simulink model "Gjennomstrommingsvarme"  (R2025b)
settings: Solver=ode45  StartTime=0.0  StopTime=30  RelTol=1e-3
model workspace (MAT data in the model file):
  SP_Final = 40
  SP_Init = 10
  SP_StepT = 2
  Tin = 10
  q_Final = 12
  q_Init = 8
  q_Lmin = 8
  q_StepT = 15
undefined symbols (not defined in the file): Kd, Ki
libraries: slpidlib x4
settings Model: Creator=Håkon  LastModifiedBy=Håkon

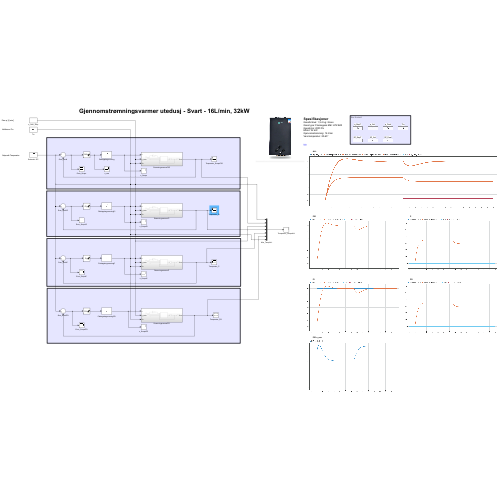
[thumbnail: Simulink's stored preview of the top-level diagram]
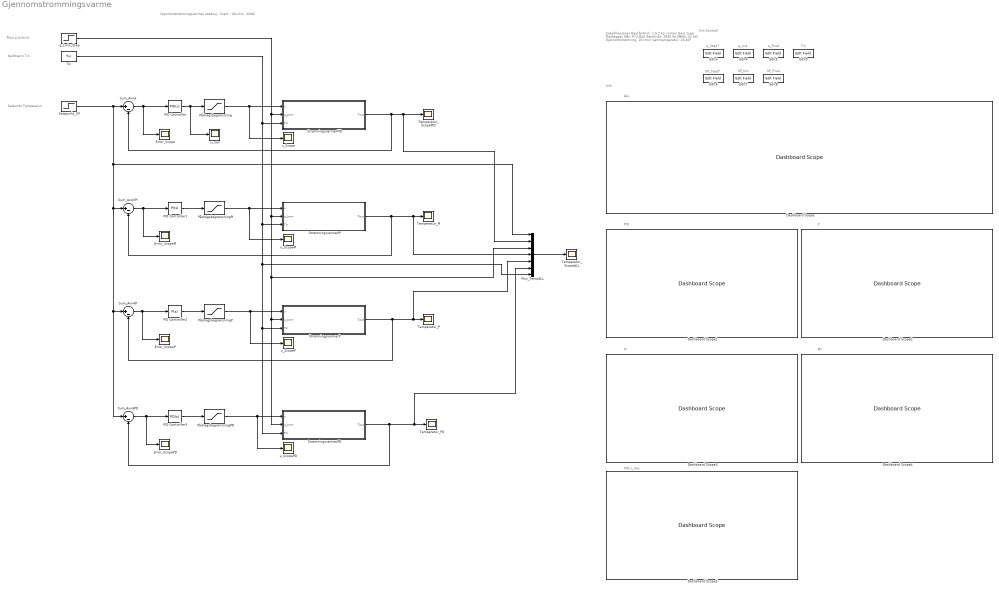
== system Gjennomstrommingsvarme ==
  note: PID
  note: Sim Kontroll
  note: Gjennomstrømningsvarmer utedusj - Svart - 16L/min, 32kW
  note: Spesifikasjoner
      | Gassforbruk: 1,5-2 kg i timen
      | Gass type: Flaskegass Mål: H72:B43
      | Gasstrykk: 2000 Pa
      | Effekt: 32 kW
      | Gjennomstrømning: 16 l/min
      | Vanntemperatur: 20-60°
  note: Link
  note: Kaldtvann Tin
  note: Flow q [L/min]
  note: Setpunkt Temperatur
  note: q_StepT
  note: q_Init
  note: q_Final
  note: SP_StepT
  note: SP_Init
  note: SP_Final
  note: Tin
  note: P
  note: PI
  note: PD
  note: ALL
  note: PID u_raw
  Dashboard Scope{,1..5} (6 alike) : DashboardScope  FontColor=[0.0, 0.0, 0.0]
  Edit{3..9} (7 alike) : EditField  LabelPosition=Hide  ShowInitialText=on  Alignment=Center
  Error_Scope : Scope
      settings: ActiveDisplayYMinimum=-1  ActiveDisplayYMaximum=1
  Error_ScopeP : Scope
      settings: ActiveDisplayYMinimum=-1  ActiveDisplayYMaximum=1  DataLoggingVariableName=ScopeData6
  Error_ScopePD : Scope
      settings: ActiveDisplayYMinimum=-1  ActiveDisplayYMaximum=1  DataLoggingVariableName=ScopeData9
  Error_ScopePI : Scope
      settings: ActiveDisplayYMinimum=-1  ActiveDisplayYMaximum=1  DataLoggingVariableName=ScopeData3
  Mux_TempALL : Mux  Inputs=7
  PID Controller : slpidlib/PID Controller  Controller=PID  Form=Parallel  TimeDomain=Continuous-time  UseExternalTs=off  SampleTime=-1  IntegratorMethod=Forward Euler  FilterMethod=Forward Euler  ControllerParametersSource=internal  P=0.03  I=0.03  UseKiTs=off  D=-0.002  UseExternalDerivativeSource=off  N=2  UseFilter=on  TunerSelectOption=Transfer Function Based (PID Tuner App)  InitialConditionSource=internal  InitialConditionForIntegrator=0  InitialConditionForFilter=0  DifferentiatorICPrevScaledInput=0  ExternalReset=none  TrackingMode=off  Kt=1  LimitOutput=on  SatLimitsSource=internal  UpperSaturationLimit=1  LowerSaturationLimit=0  LinearizeAsGain=on  AntiWindupMode=clamping  Kb=1  LimitIntegrator=off  UpperIntegratorSaturationLimit=inf  LowerIntegratorSaturationLimit=-inf  POutMin=[]  POutMax=[]  IOutMin=[]  IOutMax=[]  DOutMin=[]  DOutMax=[]  NOutMin=[]  NOutMax=[]  SumOutMin=[]  SumOutMax=[]  SaturationOutMin=[]  SaturationOutMax=[]  PParamMin=[]  PParamMax=[]  IParamMin=[]  IParamMax=[]  DParamMin=[]  DParamMax=[]  NParamMin=[]  NParamMax=[]  KbParamMin=[]  KbParamMax=[]  KtParamMin=[]  KtParamMax=[]  KbOutMin=[]  KbOutMax=[]  KtOutMin=[]  KtOutMax=[]  IntegratorOutMin=[]  IntegratorOutMax=[]  FilterOutMin=[]  FilterOutMax=[]  SumI1OutMin=[]  SumI1OutMax=[]  SumI2OutMin=[]  SumI2OutMax=[]  SumI3OutMin=[]  SumI3OutMax=[]  SumI4OutMin=[]  SumI4OutMax=[]  SumDOutMin=[]  SumDOutMax=[]  DifferentiatorOutMin=[]  DifferentiatorOutMax=[]  FilterDiffOutCoefMin=[]  FilterDiffOutCoefMax=[]  ReciprocalOutMin=[]  ReciprocalOutMax=[]  SumDenOutMin=[]  SumDenOutMax=[]  SumNumOutMin=[]  SumNumOutMax=[]  DivideOutMin=[]  DivideOutMax=[]  UdiffTsProdOutMin=[]  UdiffTsProdOutMax=[]  NTsProdOutMin=[]  NTsProdOutMax=[]  UintegralTsProdOutMin=[]  UintegralTsProdOutMax=[]  UngainTsProdOutMin=[]  UngainTsProdOutMax=[]  ClampingZeroOutDataTypeStr=Inherit: Inherit via back propagation  ClampingZeroOutMin=[]  ClampingZeroOutMax=[]  FilterDenConstantOutDataTypeStr=Inherit: Inherit via back propagation  FilterDenConstantOutMin=[]  FilterDenConstantOutMax=[]  PCopyOutDataTypeStr=Inherit: Inherit via back propagation  PCopyOutMin=[]  PCopyOutMax=[]  NCopyOutDataTypeStr=Inherit: Inherit via back propagation  NCopyOutMin=[]  NCopyOutMax=[]  IntegratorContinuousStateAttributes=''  IntegratorStateMustResolveToSignalObject=off  IntegratorRTWStateStorageClass=Auto  FilterContinuousStateAttributes=''  FilterStateMustResolveToSignalObject=off  FilterRTWStateStorageClass=Auto  ParallelPVariant=InternalParameters  IdealPVariant=Disabled  IVariant=InternalParameters  DVariant=InternalParameters  IntegratorVariant=Continuous  SatVariant=Enabled  AWVariant=ContClampingParallel  PCopyVariant=Disabled  TRVariant=Disabled  FdbkBlocksVariant=Forward  IdealPFdbkVariant=Disabled  SatFdbkVariant=Disabled  DerivativeFilterVariant=ContFilter  NVariant=InternalParameters  NCopyVariant=Disabled  FilterICVariant=InternalICsFilter  IntegratorICVariant=InternalICs  ExternalResetVariant=Disabled  TRSumVariant=Passthrough  SumFdbkVariant=Disabled  SumVariant=Sum_PID  TsampFilterVariant=InternalTs  TsampNgainVariant=Passthrough  TsampIntegralVariant=Disabled_SignalSpec  ExternalSaturationOutDataTypeStr=Inherit: Same as second input  DerivativeSourceVariant=ErrorSignal  PreIntVariant=InternalPreInt
  PID Controller1 : slpidlib/PID Controller  Controller=PI  Form=Parallel  TimeDomain=Continuous-time  UseExternalTs=off  SampleTime=-1  IntegratorMethod=Forward Euler  FilterMethod=Forward Euler  ControllerParametersSource=internal  P=0.03  I=0.03  UseKiTs=off  D=Kd  UseExternalDerivativeSource=off  N=100  UseFilter=on  TunerSelectOption=Transfer Function Based (PID Tuner App)  InitialConditionSource=internal  InitialConditionForIntegrator=0  InitialConditionForFilter=0  DifferentiatorICPrevScaledInput=0  ExternalReset=none  TrackingMode=off  Kt=1  LimitOutput=on  SatLimitsSource=internal  UpperSaturationLimit=1  LowerSaturationLimit=0  LinearizeAsGain=on  AntiWindupMode=clamping  Kb=1  LimitIntegrator=off  UpperIntegratorSaturationLimit=inf  LowerIntegratorSaturationLimit=-inf  POutMin=[]  POutMax=[]  IOutMin=[]  IOutMax=[]  DOutMin=[]  DOutMax=[]  NOutMin=[]  NOutMax=[]  SumOutMin=[]  SumOutMax=[]  SaturationOutMin=[]  SaturationOutMax=[]  PParamMin=[]  PParamMax=[]  IParamMin=[]  IParamMax=[]  DParamMin=[]  DParamMax=[]  NParamMin=[]  NParamMax=[]  KbParamMin=[]  KbParamMax=[]  KtParamMin=[]  KtParamMax=[]  KbOutMin=[]  KbOutMax=[]  KtOutMin=[]  KtOutMax=[]  IntegratorOutMin=[]  IntegratorOutMax=[]  FilterOutMin=[]  FilterOutMax=[]  SumI1OutMin=[]  SumI1OutMax=[]  SumI2OutMin=[]  SumI2OutMax=[]  SumI3OutMin=[]  SumI3OutMax=[]  SumI4OutMin=[]  SumI4OutMax=[]  SumDOutMin=[]  SumDOutMax=[]  DifferentiatorOutMin=[]  DifferentiatorOutMax=[]  FilterDiffOutCoefMin=[]  FilterDiffOutCoefMax=[]  ReciprocalOutMin=[]  ReciprocalOutMax=[]  SumDenOutMin=[]  SumDenOutMax=[]  SumNumOutMin=[]  SumNumOutMax=[]  DivideOutMin=[]  DivideOutMax=[]  UdiffTsProdOutMin=[]  UdiffTsProdOutMax=[]  NTsProdOutMin=[]  NTsProdOutMax=[]  UintegralTsProdOutMin=[]  UintegralTsProdOutMax=[]  UngainTsProdOutMin=[]  UngainTsProdOutMax=[]  ClampingZeroOutDataTypeStr=Inherit: Inherit via back propagation  ClampingZeroOutMin=[]  ClampingZeroOutMax=[]  FilterDenConstantOutDataTypeStr=Inherit: Inherit via back propagation  FilterDenConstantOutMin=[]  FilterDenConstantOutMax=[]  PCopyOutDataTypeStr=Inherit: Inherit via back propagation  PCopyOutMin=[]  PCopyOutMax=[]  NCopyOutDataTypeStr=Inherit: Inherit via back propagation  NCopyOutMin=[]  NCopyOutMax=[]  IntegratorContinuousStateAttributes=''  IntegratorStateMustResolveToSignalObject=off  IntegratorRTWStateStorageClass=Auto  FilterContinuousStateAttributes=''  FilterStateMustResolveToSignalObject=off  FilterRTWStateStorageClass=Auto  ParallelPVariant=InternalParameters  IdealPVariant=Disabled  IVariant=InternalParameters  DVariant=Disabled  IntegratorVariant=Continuous  SatVariant=Enabled  AWVariant=ContClampingParallel  PCopyVariant=Disabled  TRVariant=Disabled  FdbkBlocksVariant=Forward  IdealPFdbkVariant=Disabled  SatFdbkVariant=Disabled  DerivativeFilterVariant=Disabled  NVariant=Disabled  NCopyVariant=Disabled_SignalSpec  FilterICVariant=Disabled  IntegratorICVariant=InternalICs  ExternalResetVariant=Disabled  TRSumVariant=Passthrough  SumFdbkVariant=Disabled  SumVariant=Sum_PI  TsampFilterVariant=InternalTs  TsampNgainVariant=Passthrough  TsampIntegralVariant=Disabled_SignalSpec  ExternalSaturationOutDataTypeStr=Inherit: Same as second input  DerivativeSourceVariant=Disabled  PreIntVariant=InternalPreInt
  PID Controller2 : slpidlib/PID Controller  Controller=P  Form=Parallel  TimeDomain=Continuous-time  UseExternalTs=off  SampleTime=-1  IntegratorMethod=Forward Euler  FilterMethod=Forward Euler  ControllerParametersSource=internal  P=0.03  I=Ki  UseKiTs=off  D=Kd  UseExternalDerivativeSource=off  N=100  UseFilter=on  TunerSelectOption=Transfer Function Based (PID Tuner App)  InitialConditionSource=internal  InitialConditionForIntegrator=0  InitialConditionForFilter=0  DifferentiatorICPrevScaledInput=0  ExternalReset=none  TrackingMode=off  Kt=1  LimitOutput=on  SatLimitsSource=internal  UpperSaturationLimit=1  LowerSaturationLimit=0  LinearizeAsGain=on  AntiWindupMode=clamping  Kb=1  LimitIntegrator=off  UpperIntegratorSaturationLimit=inf  LowerIntegratorSaturationLimit=-inf  POutMin=[]  POutMax=[]  IOutMin=[]  IOutMax=[]  DOutMin=[]  DOutMax=[]  NOutMin=[]  NOutMax=[]  SumOutMin=[]  SumOutMax=[]  SaturationOutMin=[]  SaturationOutMax=[]  PParamMin=[]  PParamMax=[]  IParamMin=[]  IParamMax=[]  DParamMin=[]  DParamMax=[]  NParamMin=[]  NParamMax=[]  KbParamMin=[]  KbParamMax=[]  KtParamMin=[]  KtParamMax=[]  KbOutMin=[]  KbOutMax=[]  KtOutMin=[]  KtOutMax=[]  IntegratorOutMin=[]  IntegratorOutMax=[]  FilterOutMin=[]  FilterOutMax=[]  SumI1OutMin=[]  SumI1OutMax=[]  SumI2OutMin=[]  SumI2OutMax=[]  SumI3OutMin=[]  SumI3OutMax=[]  SumI4OutMin=[]  SumI4OutMax=[]  SumDOutMin=[]  SumDOutMax=[]  DifferentiatorOutMin=[]  DifferentiatorOutMax=[]  FilterDiffOutCoefMin=[]  FilterDiffOutCoefMax=[]  ReciprocalOutMin=[]  ReciprocalOutMax=[]  SumDenOutMin=[]  SumDenOutMax=[]  SumNumOutMin=[]  SumNumOutMax=[]  DivideOutMin=[]  DivideOutMax=[]  UdiffTsProdOutMin=[]  UdiffTsProdOutMax=[]  NTsProdOutMin=[]  NTsProdOutMax=[]  UintegralTsProdOutMin=[]  UintegralTsProdOutMax=[]  UngainTsProdOutMin=[]  UngainTsProdOutMax=[]  ClampingZeroOutDataTypeStr=Inherit: Inherit via back propagation  ClampingZeroOutMin=[]  ClampingZeroOutMax=[]  FilterDenConstantOutDataTypeStr=Inherit: Inherit via back propagation  FilterDenConstantOutMin=[]  FilterDenConstantOutMax=[]  PCopyOutDataTypeStr=Inherit: Inherit via back propagation  PCopyOutMin=[]  PCopyOutMax=[]  NCopyOutDataTypeStr=Inherit: Inherit via back propagation  NCopyOutMin=[]  NCopyOutMax=[]  IntegratorContinuousStateAttributes=''  IntegratorStateMustResolveToSignalObject=off  IntegratorRTWStateStorageClass=Auto  FilterContinuousStateAttributes=''  FilterStateMustResolveToSignalObject=off  FilterRTWStateStorageClass=Auto  ParallelPVariant=InternalParameters  IdealPVariant=Disabled  IVariant=Disabled  DVariant=Disabled  IntegratorVariant=Disabled  SatVariant=Enabled  AWVariant=Disabled  PCopyVariant=Disabled  TRVariant=Disabled  FdbkBlocksVariant=Forward  IdealPFdbkVariant=Disabled  SatFdbkVariant=Disabled  DerivativeFilterVariant=Disabled  NVariant=Disabled  NCopyVariant=Disabled_SignalSpec  FilterICVariant=Disabled  IntegratorICVariant=Disabled  ExternalResetVariant=Disabled  TRSumVariant=Passthrough  SumFdbkVariant=Disabled  SumVariant=Passthrough_P  TsampFilterVariant=InternalTs  TsampNgainVariant=Passthrough  TsampIntegralVariant=Disabled_SignalSpec  ExternalSaturationOutDataTypeStr=Inherit: Same as second input  DerivativeSourceVariant=Disabled  PreIntVariant=InternalPreInt
  PID Controller3 : slpidlib/PID Controller  Controller=PD  Form=Parallel  TimeDomain=Continuous-time  UseExternalTs=off  SampleTime=-1  IntegratorMethod=Forward Euler  FilterMethod=Forward Euler  ControllerParametersSource=internal  P=0.03  I=Ki  UseKiTs=off  D=-0.002  UseExternalDerivativeSource=off  N=2  UseFilter=on  TunerSelectOption=Transfer Function Based (PID Tuner App)  InitialConditionSource=internal  InitialConditionForIntegrator=0  InitialConditionForFilter=0  DifferentiatorICPrevScaledInput=0  ExternalReset=none  TrackingMode=off  Kt=1  LimitOutput=on  SatLimitsSource=internal  UpperSaturationLimit=1  LowerSaturationLimit=0  LinearizeAsGain=on  AntiWindupMode=clamping  Kb=1  LimitIntegrator=off  UpperIntegratorSaturationLimit=inf  LowerIntegratorSaturationLimit=-inf  POutMin=[]  POutMax=[]  IOutMin=[]  IOutMax=[]  DOutMin=[]  DOutMax=[]  NOutMin=[]  NOutMax=[]  SumOutMin=[]  SumOutMax=[]  SaturationOutMin=[]  SaturationOutMax=[]  PParamMin=[]  PParamMax=[]  IParamMin=[]  IParamMax=[]  DParamMin=[]  DParamMax=[]  NParamMin=[]  NParamMax=[]  KbParamMin=[]  KbParamMax=[]  KtParamMin=[]  KtParamMax=[]  KbOutMin=[]  KbOutMax=[]  KtOutMin=[]  KtOutMax=[]  IntegratorOutMin=[]  IntegratorOutMax=[]  FilterOutMin=[]  FilterOutMax=[]  SumI1OutMin=[]  SumI1OutMax=[]  SumI2OutMin=[]  SumI2OutMax=[]  SumI3OutMin=[]  SumI3OutMax=[]  SumI4OutMin=[]  SumI4OutMax=[]  SumDOutMin=[]  SumDOutMax=[]  DifferentiatorOutMin=[]  DifferentiatorOutMax=[]  FilterDiffOutCoefMin=[]  FilterDiffOutCoefMax=[]  ReciprocalOutMin=[]  ReciprocalOutMax=[]  SumDenOutMin=[]  SumDenOutMax=[]  SumNumOutMin=[]  SumNumOutMax=[]  DivideOutMin=[]  DivideOutMax=[]  UdiffTsProdOutMin=[]  UdiffTsProdOutMax=[]  NTsProdOutMin=[]  NTsProdOutMax=[]  UintegralTsProdOutMin=[]  UintegralTsProdOutMax=[]  UngainTsProdOutMin=[]  UngainTsProdOutMax=[]  ClampingZeroOutDataTypeStr=Inherit: Inherit via back propagation  ClampingZeroOutMin=[]  ClampingZeroOutMax=[]  FilterDenConstantOutDataTypeStr=Inherit: Inherit via back propagation  FilterDenConstantOutMin=[]  FilterDenConstantOutMax=[]  PCopyOutDataTypeStr=Inherit: Inherit via back propagation  PCopyOutMin=[]  PCopyOutMax=[]  NCopyOutDataTypeStr=Inherit: Inherit via back propagation  NCopyOutMin=[]  NCopyOutMax=[]  IntegratorContinuousStateAttributes=''  IntegratorStateMustResolveToSignalObject=off  IntegratorRTWStateStorageClass=Auto  FilterContinuousStateAttributes=''  FilterStateMustResolveToSignalObject=off  FilterRTWStateStorageClass=Auto  ParallelPVariant=InternalParameters  IdealPVariant=Disabled  IVariant=Disabled  DVariant=InternalParameters  IntegratorVariant=Disabled  SatVariant=Enabled  AWVariant=Disabled  PCopyVariant=Disabled  TRVariant=Disabled  FdbkBlocksVariant=Forward  IdealPFdbkVariant=Disabled  SatFdbkVariant=Disabled  DerivativeFilterVariant=ContFilter  NVariant=InternalParameters  NCopyVariant=Disabled  FilterICVariant=InternalICsFilter  IntegratorICVariant=Disabled  ExternalResetVariant=Disabled  TRSumVariant=Passthrough  SumFdbkVariant=Disabled  SumVariant=Sum_PD  TsampFilterVariant=InternalTs  TsampNgainVariant=Passthrough  TsampIntegralVariant=Disabled_SignalSpec  ExternalSaturationOutDataTypeStr=Inherit: Same as second input  DerivativeSourceVariant=ErrorSignal  PreIntVariant=InternalPreInt
  Pådragsbegrensning : Saturate  UpperLimit=1  LowerLimit=0
  PådragsbegrensningP : Saturate  UpperLimit=1  LowerLimit=0
  PådragsbegrensningPD : Saturate  UpperLimit=1  LowerLimit=0
  PådragsbegrensningPI : Saturate  UpperLimit=1  LowerLimit=0
  Settpunkt_SP : Step  Time=SP_StepT  Before=SP_Init  After=SP_Final  SampleTime=0
  StrømningsvarmerP : Subsystem
  StrømningsvarmerPD : Subsystem
  StrømningsvarmerPI : Subsystem
  StrømningsvarmerPID : Subsystem
  Sum_Avvik : Sum  Inputs=|+-
  Sum_AvvikP : Sum  Inputs=|+-
  Sum_AvvikPD : Sum  Inputs=|+-
  Sum_AvvikPI : Sum  Inputs=|+-
  Temperatur_P : Scope
      settings: ActiveDisplayYMinimum=6.4940957211164019  ActiveDisplayYMaximum=41.55313850995239  DataLoggingVariableName=ScopeData7
  Temperatur_PD : Scope
      settings: ActiveDisplayYMinimum=7.7892303218856442  ActiveDisplayYMaximum=29.89692710302921  DataLoggingVariableName=ScopeData10
  Temperatur_PI : Scope
      settings: ActiveDisplayYMinimum=6.0133689334322051  ActiveDisplayYMaximum=45.879679599110162  DataLoggingVariableName=ScopeData4
  Temperatur_ScopeALL : Scope
      settings: ActiveDisplayYMinimum=-19.252072166409661  ActiveDisplayYMaximum=81.341690384246078  DataLoggingVariableName=ScopeData12
  Temperatur_ScopePID : Scope
      settings: ActiveDisplayYMinimum=6.00522530086716  ActiveDisplayYMaximum=45.952972292195568
  Tin : Constant  Value=Tin
  q_Lmin_Step : Step  Time=q_StepT  Before=q_Init  After=q_Final  SampleTime=0
  u_Scope : Scope
      settings: ActiveDisplayYMinimum=-1  ActiveDisplayYMaximum=1  DataLoggingVariableName=ScopeData2
  u_ScopeP : Scope
      settings: ActiveDisplayYMinimum=-1  ActiveDisplayYMaximum=1  DataLoggingVariableName=ScopeData8
  u_ScopePD : Scope
      settings: ActiveDisplayYMinimum=-1  ActiveDisplayYMaximum=1  DataLoggingVariableName=ScopeData11
  u_ScopePI : Scope
      settings: ActiveDisplayYMinimum=-1  ActiveDisplayYMaximum=1  DataLoggingVariableName=ScopeData5
  u_raw : Scope
      settings: ActiveDisplayYMinimum=-1  ActiveDisplayYMaximum=1  DataLoggingVariableName=ScopeData13
  wires:
  Sum_Avvik/1 -> PID Controller/1, Error_Scope/1
  Pådragsbegrensning/1 -> u_Scope/1, StrømningsvarmerPID/1(u)
  PID Controller/1 -> u_raw/1, Pådragsbegrensning/1
  PådragsbegrensningPI/1 -> StrømningsvarmerPI/1(u), u_ScopePI/1
  Sum_AvvikPI/1 -> PID Controller1/1, Error_ScopePI/1
  StrømningsvarmerPI/1(Tout) -> Mux_TempALL/4, Temperatur_PI/1, Sum_AvvikPI/2
  PID Controller2/1 -> PådragsbegrensningP/1
  StrømningsvarmerP/1(Tout) -> Mux_TempALL/5, Temperatur_P/1, Sum_AvvikP/2
  PådragsbegrensningP/1 -> u_ScopeP/1, StrømningsvarmerP/1(u)
  Sum_AvvikP/1 -> Error_ScopeP/1, PID Controller2/1
  q_Lmin_Step/1 -> Mux_TempALL/3, StrømningsvarmerPD/2(q_Lmin), StrømningsvarmerP/2(q_Lmin), StrømningsvarmerPI/2(q_Lmin), StrømningsvarmerPID/2(q_Lmin)
  Tin/1 -> StrømningsvarmerPID/3(Tin), Mux_TempALL/7, StrømningsvarmerP/3(Tin), StrømningsvarmerPD/3(Tin), StrømningsvarmerPI/3(Tin)
  Settpunkt_SP/1 -> Mux_TempALL/1, Sum_AvvikPI/1, Sum_AvvikPD/1, Sum_AvvikP/1, Sum_Avvik/1
  PID Controller3/1 -> PådragsbegrensningPD/1
  StrømningsvarmerPD/1(Tout) -> Mux_TempALL/6, Temperatur_PD/1, Sum_AvvikPD/2
  PådragsbegrensningPD/1 -> StrømningsvarmerPD/1(u), u_ScopePD/1
  Mux_TempALL/1 -> Temperatur_ScopeALL/1
  Sum_AvvikPD/1 -> Error_ScopePD/1, PID Controller3/1
  PID Controller1/1 -> PådragsbegrensningPI/1
  StrømningsvarmerPID/1(Tout) -> Mux_TempALL/2, Temperatur_ScopePID/1, Sum_Avvik/2

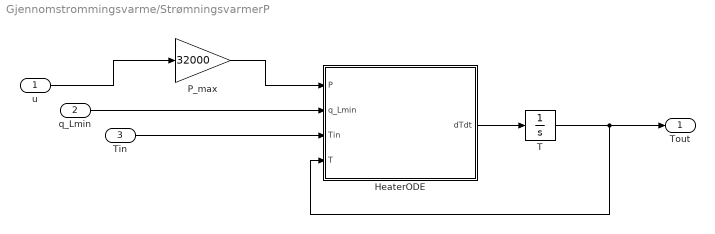
== system Gjennomstrommingsvarme/StrømningsvarmerP ==
  u : Inport
  q_Lmin : Inport  Port=2
  Tin : Inport  Port=3
  HeaterODE : MATLAB Function  TreatAsAtomicUnit=on
  P_max : Gain  Gain=32000
  T : Integrator  InitialCondition=Tin
  Tout : Outport
  wires:
  q_Lmin/1 -> HeaterODE/2(q_Lmin)
  Tin/1 -> HeaterODE/3(Tin)
  HeaterODE/1(dTdt) -> T/1
  T/1 -> Tout/1, HeaterODE/4(T)
  P_max/1 -> HeaterODE/1(P)
  u/1 -> P_max/1

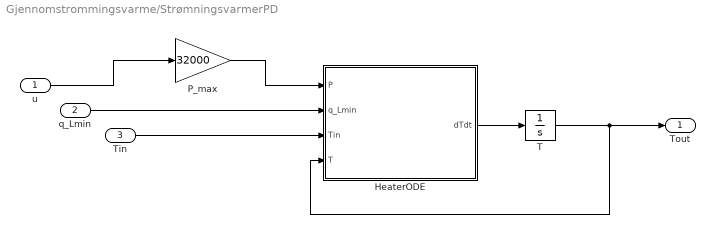
== system Gjennomstrommingsvarme/StrømningsvarmerPD ==
  u : Inport
  q_Lmin : Inport  Port=2
  Tin : Inport  Port=3
  HeaterODE : MATLAB Function  TreatAsAtomicUnit=on
  P_max : Gain  Gain=32000
  T : Integrator  InitialCondition=Tin
  Tout : Outport
  wires:
  q_Lmin/1 -> HeaterODE/2(q_Lmin)
  Tin/1 -> HeaterODE/3(Tin)
  HeaterODE/1(dTdt) -> T/1
  T/1 -> Tout/1, HeaterODE/4(T)
  P_max/1 -> HeaterODE/1(P)
  u/1 -> P_max/1

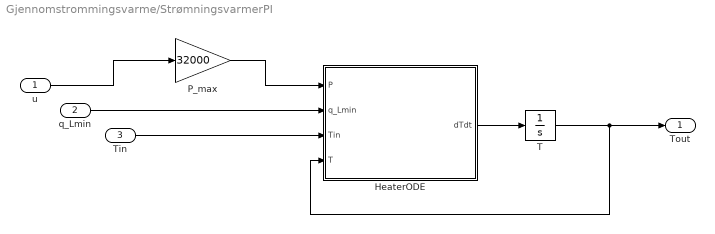
== system Gjennomstrommingsvarme/StrømningsvarmerPI ==
  u : Inport
  q_Lmin : Inport  Port=2
  Tin : Inport  Port=3
  HeaterODE : MATLAB Function  TreatAsAtomicUnit=on
  P_max : Gain  Gain=32000
  T : Integrator  InitialCondition=Tin
  Tout : Outport
  wires:
  q_Lmin/1 -> HeaterODE/2(q_Lmin)
  Tin/1 -> HeaterODE/3(Tin)
  HeaterODE/1(dTdt) -> T/1
  T/1 -> Tout/1, HeaterODE/4(T)
  P_max/1 -> HeaterODE/1(P)
  u/1 -> P_max/1

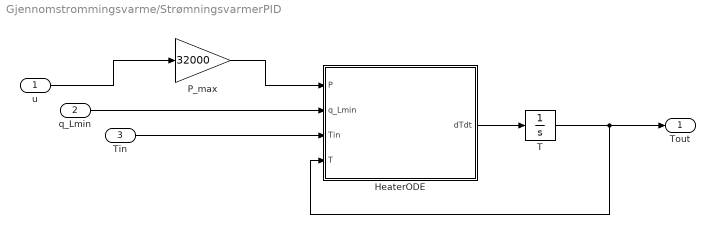
== system Gjennomstrommingsvarme/StrømningsvarmerPID ==
  u : Inport
  q_Lmin : Inport  Port=2
  Tin : Inport  Port=3
  HeaterODE : MATLAB Function  TreatAsAtomicUnit=on
  P_max : Gain  Gain=32000
  T : Integrator  InitialCondition=Tin
  Tout : Outport
  wires:
  q_Lmin/1 -> HeaterODE/2(q_Lmin)
  Tin/1 -> HeaterODE/3(Tin)
  HeaterODE/1(dTdt) -> T/1
  T/1 -> Tout/1, HeaterODE/4(T)
  P_max/1 -> HeaterODE/1(P)
  u/1 -> P_max/1

== matlab function Gjennomstrommingsvarme/StrømningsvarmerPI/HeaterODE ==
  data: P input; dTdt output; q_Lmin input; Tin input; T input
function dTdt = HeaterODE(P, q_Lmin, Tin, T)
% HeaterODE - Forbedret modell for gass-gjennomstroemningsvarmer
% Utendoersdusj 32kW
%
% Denne versjonen bruker SKALAR T (vanntemperatur) slik at den fungerer
% direkte med eksisterende Simulink-modell uten endringer i integrator
% eller signalruting.
%
% Forbedringer vs. original:
%   - Forbrenningsvirkningsgrad (eta = 85%)
%   - Varmetap til omgivelser (UA_ma)
%   - Effektiv varmeovergang justert for gjennomstroemningsvarmer
%
% Referanser:
%   [1] Incropera et al., "Fundamentals of Heat and Mass Transfer", 7e, Wiley, 2011.
%   [2] Cengel, "Heat Transfer: A Practical Approach", 2e, McGraw-Hill, 2003.
%
% Innganger:
%   P       - Varmeeffekt fra brenner [W] (0 til 32000 W)
%   q_Lmin  - Volumstroem vann [L/min] (maks 16 L/min)
%   Tin     - Innloepstemperatur vann [degC]
%   T       - Utloepstemperatur vann [degC] (tilbakekobling, skalar)
%
% Utgang:
%   dTdt    - Temperaturendring [degC/s] (skalar)

% =====================================================================
%  VANNETS EGENSKAPER [1, Tabell A.6]
% =====================================================================
cp    = 4186;          % Spesifikk varmekapasitet vann [J/(kg*K)]
rho   = 1.0;           % Tetthet vann [kg/L]

% =====================================================================
%  FORBRENNINGSEFFEKTIVITET [2, Kap. 13]
% =====================================================================
eta   = 0.85;          % Virkningsgrad gassbrenner (85%)

% =====================================================================
%  MASSESTROEMM
% =====================================================================
mdot  = (q_Lmin / 60) * rho;  % [kg/s]

% =====================================================================
%  VARMEVEKSLER - tilpasset gjennomstroemningsvarmer
% =====================================================================
% Kompakt kobberspiral med direkte flamme.
% Lite vannvolum gir kort oppholdstid (ca. 2 sekunder ved 8 L/min).
V     = 0.25;          % Vannvolum i veksler [L]
C     = V * rho * cp;  % Termisk kapasitet vann [J/K] = 1046.5

% =====================================================================
%  VARMETAP TIL OMGIVELSER
% =====================================================================
UA_loss = 10;          % Konduktans til omgivelser [W/K]
T_amb   = 10;          % Omgivelsestemperatur [degC]
Q_loss  = UA_loss * (T - T_amb);  % Varmetap [W]

% =====================================================================
%  ENERGIBALANSE
% =====================================================================
%  C * dT/dt = eta*P - Q_loss + mdot*cp*(Tin - T)
%
%  Ledd:
%    eta*P              : Effektiv varme fra gassforbrenning [W]
%    Q_loss             : Varmetap til omgivelser [W]
%    mdot*cp*(Tin - T)  : Netto varme fra vannstroemmen [W]

dTdt = (eta * P - Q_loss + mdot * cp * (Tin - T)) / C;

end

== matlab function Gjennomstrommingsvarme/StrømningsvarmerPID/HeaterODE ==
  data: P input; dTdt output; q_Lmin input; Tin input; T input
function dTdt = HeaterODE(P, q_Lmin, Tin, T)
% HeaterODE - Forbedret modell for gass-gjennomstroemningsvarmer
% Utendoersdusj 32kW
%
% Denne versjonen bruker SKALAR T (vanntemperatur) slik at den fungerer
% direkte med eksisterende Simulink-modell uten endringer i integrator
% eller signalruting.
%
% Forbedringer vs. original:
%   - Forbrenningsvirkningsgrad (eta = 85%)
%   - Varmetap til omgivelser (UA_ma)
%   - Effektiv varmeovergang justert for gjennomstroemningsvarmer
%
% Referanser:
%   [1] Incropera et al., "Fundamentals of Heat and Mass Transfer", 7e, Wiley, 2011.
%   [2] Cengel, "Heat Transfer: A Practical Approach", 2e, McGraw-Hill, 2003.
%
% Innganger:
%   P       - Varmeeffekt fra brenner [W] (0 til 32000 W)
%   q_Lmin  - Volumstroem vann [L/min] (maks 16 L/min)
%   Tin     - Innloepstemperatur vann [degC]
%   T       - Utloepstemperatur vann [degC] (tilbakekobling, skalar)
%
% Utgang:
%   dTdt    - Temperaturendring [degC/s] (skalar)

% =====================================================================
%  VANNETS EGENSKAPER [1, Tabell A.6]
% =====================================================================
cp    = 4186;          % Spesifikk varmekapasitet vann [J/(kg*K)]
rho   = 1.0;           % Tetthet vann [kg/L]

% =====================================================================
%  FORBRENNINGSEFFEKTIVITET [2, Kap. 13]
% =====================================================================
eta   = 0.85;          % Virkningsgrad gassbrenner (85%)

% =====================================================================
%  MASSESTROEMM
% =====================================================================
mdot  = (q_Lmin / 60) * rho;  % [kg/s]

% =====================================================================
%  VARMEVEKSLER - tilpasset gjennomstroemningsvarmer
% =====================================================================
% Kompakt kobberspiral med direkte flamme.
% Lite vannvolum gir kort oppholdstid (ca. 2 sekunder ved 8 L/min).
V     = 0.25;          % Vannvolum i veksler [L]
C     = V * rho * cp;  % Termisk kapasitet vann [J/K] = 1046.5

% =====================================================================
%  VARMETAP TIL OMGIVELSER
% =====================================================================
UA_loss = 10;          % Konduktans til omgivelser [W/K]
T_amb   = 10;          % Omgivelsestemperatur [degC]
Q_loss  = UA_loss * (T - T_amb);  % Varmetap [W]

% =====================================================================
%  ENERGIBALANSE
% =====================================================================
%  C * dT/dt = eta*P - Q_loss + mdot*cp*(Tin - T)
%
%  Ledd:
%    eta*P              : Effektiv varme fra gassforbrenning [W]
%    Q_loss             : Varmetap til omgivelser [W]
%    mdot*cp*(Tin - T)  : Netto varme fra vannstroemmen [W]

dTdt = (eta * P - Q_loss + mdot * cp * (Tin - T)) / C;

end

== matlab function Gjennomstrommingsvarme/StrømningsvarmerP/HeaterODE ==
  data: P input; dTdt output; q_Lmin input; Tin input; T input
function dTdt = HeaterODE(P, q_Lmin, Tin, T)
% HeaterODE - Forbedret modell for gass-gjennomstroemningsvarmer
% Utendoersdusj 32kW
%
% Denne versjonen bruker SKALAR T (vanntemperatur) slik at den fungerer
% direkte med eksisterende Simulink-modell uten endringer i integrator
% eller signalruting.
%
% Forbedringer vs. original:
%   - Forbrenningsvirkningsgrad (eta = 85%)
%   - Varmetap til omgivelser (UA_ma)
%   - Effektiv varmeovergang justert for gjennomstroemningsvarmer
%
% Referanser:
%   [1] Incropera et al., "Fundamentals of Heat and Mass Transfer", 7e, Wiley, 2011.
%   [2] Cengel, "Heat Transfer: A Practical Approach", 2e, McGraw-Hill, 2003.
%
% Innganger:
%   P       - Varmeeffekt fra brenner [W] (0 til 32000 W)
%   q_Lmin  - Volumstroem vann [L/min] (maks 16 L/min)
%   Tin     - Innloepstemperatur vann [degC]
%   T       - Utloepstemperatur vann [degC] (tilbakekobling, skalar)
%
% Utgang:
%   dTdt    - Temperaturendring [degC/s] (skalar)

% =====================================================================
%  VANNETS EGENSKAPER [1, Tabell A.6]
% =====================================================================
cp    = 4186;          % Spesifikk varmekapasitet vann [J/(kg*K)]
rho   = 1.0;           % Tetthet vann [kg/L]

% =====================================================================
%  FORBRENNINGSEFFEKTIVITET [2, Kap. 13]
% =====================================================================
eta   = 0.85;          % Virkningsgrad gassbrenner (85%)

% =====================================================================
%  MASSESTROEMM
% =====================================================================
mdot  = (q_Lmin / 60) * rho;  % [kg/s]

% =====================================================================
%  VARMEVEKSLER - tilpasset gjennomstroemningsvarmer
% =====================================================================
% Kompakt kobberspiral med direkte flamme.
% Lite vannvolum gir kort oppholdstid (ca. 2 sekunder ved 8 L/min).
V     = 0.25;          % Vannvolum i veksler [L]
C     = V * rho * cp;  % Termisk kapasitet vann [J/K] = 1046.5

% =====================================================================
%  VARMETAP TIL OMGIVELSER
% =====================================================================
UA_loss = 10;          % Konduktans til omgivelser [W/K]
T_amb   = 10;          % Omgivelsestemperatur [degC]
Q_loss  = UA_loss * (T - T_amb);  % Varmetap [W]

% =====================================================================
%  ENERGIBALANSE
% =====================================================================
%  C * dT/dt = eta*P - Q_loss + mdot*cp*(Tin - T)
%
%  Ledd:
%    eta*P              : Effektiv varme fra gassforbrenning [W]
%    Q_loss             : Varmetap til omgivelser [W]
%    mdot*cp*(Tin - T)  : Netto varme fra vannstroemmen [W]

dTdt = (eta * P - Q_loss + mdot * cp * (Tin - T)) / C;

end

== matlab function Gjennomstrommingsvarme/StrømningsvarmerPD/HeaterODE ==
  data: P input; dTdt output; q_Lmin input; Tin input; T input
function dTdt = HeaterODE(P, q_Lmin, Tin, T)
% HeaterODE - Forbedret modell for gass-gjennomstroemningsvarmer
% Utendoersdusj 32kW
%
% Denne versjonen bruker SKALAR T (vanntemperatur) slik at den fungerer
% direkte med eksisterende Simulink-modell uten endringer i integrator
% eller signalruting.
%
% Forbedringer vs. original:
%   - Forbrenningsvirkningsgrad (eta = 85%)
%   - Varmetap til omgivelser (UA_ma)
%   - Effektiv varmeovergang justert for gjennomstroemningsvarmer
%
% Referanser:
%   [1] Incropera et al., "Fundamentals of Heat and Mass Transfer", 7e, Wiley, 2011.
%   [2] Cengel, "Heat Transfer: A Practical Approach", 2e, McGraw-Hill, 2003.
%
% Innganger:
%   P       - Varmeeffekt fra brenner [W] (0 til 32000 W)
%   q_Lmin  - Volumstroem vann [L/min] (maks 16 L/min)
%   Tin     - Innloepstemperatur vann [degC]
%   T       - Utloepstemperatur vann [degC] (tilbakekobling, skalar)
%
% Utgang:
%   dTdt    - Temperaturendring [degC/s] (skalar)

% =====================================================================
%  VANNETS EGENSKAPER [1, Tabell A.6]
% =====================================================================
cp    = 4186;          % Spesifikk varmekapasitet vann [J/(kg*K)]
rho   = 1.0;           % Tetthet vann [kg/L]

% =====================================================================
%  FORBRENNINGSEFFEKTIVITET [2, Kap. 13]
% =====================================================================
eta   = 0.85;          % Virkningsgrad gassbrenner (85%)

% =====================================================================
%  MASSESTROEMM
% =====================================================================
mdot  = (q_Lmin / 60) * rho;  % [kg/s]

% =====================================================================
%  VARMEVEKSLER - tilpasset gjennomstroemningsvarmer
% =====================================================================
% Kompakt kobberspiral med direkte flamme.
% Lite vannvolum gir kort oppholdstid (ca. 2 sekunder ved 8 L/min).
V     = 0.25;          % Vannvolum i veksler [L]
C     = V * rho * cp;  % Termisk kapasitet vann [J/K] = 1046.5

% =====================================================================
%  VARMETAP TIL OMGIVELSER
% =====================================================================
UA_loss = 10;          % Konduktans til omgivelser [W/K]
T_amb   = 10;          % Omgivelsestemperatur [degC]
Q_loss  = UA_loss * (T - T_amb);  % Varmetap [W]

% =====================================================================
%  ENERGIBALANSE
% =====================================================================
%  C * dT/dt = eta*P - Q_loss + mdot*cp*(Tin - T)
%
%  Ledd:
%    eta*P              : Effektiv varme fra gassforbrenning [W]
%    Q_loss             : Varmetap til omgivelser [W]
%    mdot*cp*(Tin - T)  : Netto varme fra vannstroemmen [W]

dTdt = (eta * P - Q_loss + mdot * cp * (Tin - T)) / C;

end
